simulink model "Task_8_2"  (R2015a)
settings: Solver=ode45  StartTime=0.0  StopTime=10.0  RelTol=1e-3
settings Model: Creator=acer  LastModifiedBy=acer

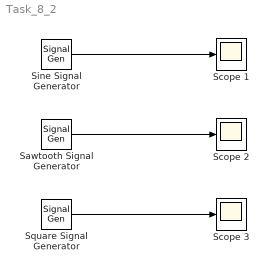
== system Task_8_2 ==
  Sawtooth Signal Generator : SignalGenerator  WaveForm=sawtooth  Units=rad/sec
  Scope 1 : Scope
  Scope 2 : Scope
      settings: SaveName=ScopeData2
  Scope 3 : Scope
  Sine Signal Generator : SignalGenerator  Units=rad/sec
  Square Signal Generator : SignalGenerator  WaveForm=square  Units=rad/sec
  wires:
  Sine Signal Generator/1 -> Scope 1/1
  Sawtooth Signal Generator/1 -> Scope 2/1
  Square Signal Generator/1 -> Scope 3/1
